simulink model "ME4391L_LAB2_Goulenko_P1"  (R2021b)
settings: Solver=FixedStepAuto  StartTime=0.0  StopTime=10.0  FixedStep=.01  RelTol=1e-3
values from neighbouring files (symbols this model uses):
  a = 2    [AndyVoLab2.m]    (also in ME4391L_LAB2_Goulenko_P2.m)
  b = 3    [AndyVoLab2.m]    (also in ME4391L_LAB2_Goulenko_P2.m)
  c = 0.25    [AndyVoLab2.m]    (also in ME4391L_LAB2_Goulenko_P2.m)
  d = 1 * 2*pi    (= 6.28318530718)    [AndyVoLab2.m]    (also in ME4391L_LAB2_Goulenko_P2.m)
settings Model: Creator=gkgoulenko  LastModifiedBy=gkgoulenko
settings DataIOCC: ReturnWorkspaceOutputs=off

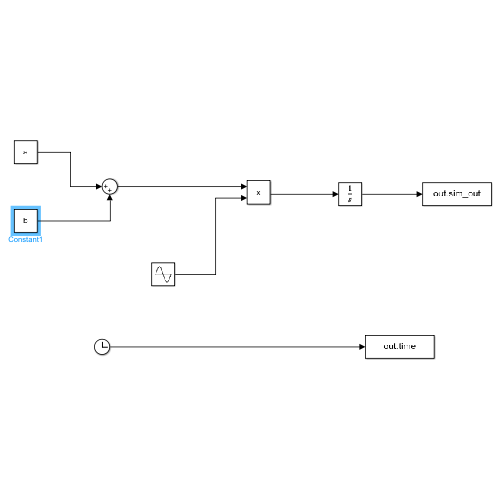
[thumbnail: Simulink's stored preview of the top-level diagram]
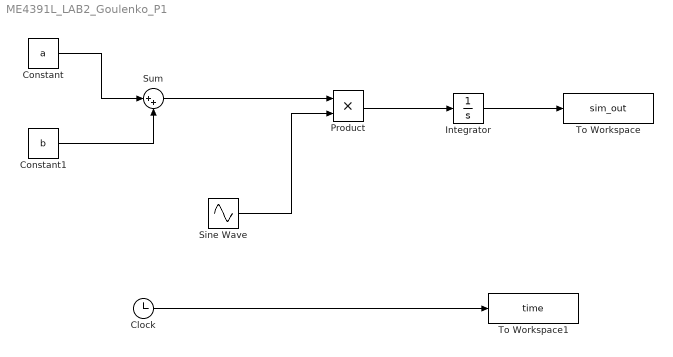
== system ME4391L_LAB2_Goulenko_P1 ==
  Clock : Clock
  Constant : Constant  Value=a
  Constant1 : Constant  Value=b
  Integrator : Integrator
  Product : Product
  Sine Wave : Sin  Amplitude=c  Frequency=d  SampleTime=0
  Sum : Sum  Inputs=|++
  To Workspace : ToWorkspace  VariableName=sim_out  SampleTime=-1
      settings: Save2DSignal=2-D array (concatenate along first dimension)
  To Workspace1 : ToWorkspace  VariableName=time  SampleTime=-1
      settings: Save2DSignal=2-D array (concatenate along first dimension)
  wires:
  Constant1/1 -> Sum/2
  Constant/1 -> Sum/1
  Sum/1 -> Product/1
  Sine Wave/1 -> Product/2
  Product/1 -> Integrator/1
  Integrator/1 -> To Workspace/1
  Clock/1 -> To Workspace1/1
